simulink model "servo_real"  (Simulink 6.2)
settings: Solver=ode45  StartTime=0.0  StopTime=10  RelTol=1e-3
PreLoadFcn:
  | init_servo
libraries: cstblocks x2, simulink x2
settings Model: Creator=f96to  LastModifiedBy=toivo  ExtModeAutoUpdateStatusClock=off
settings OptimizationCC: BlockReduction=off  BooleanDataType=off
settings HardwareCC: TargetUnknown=on

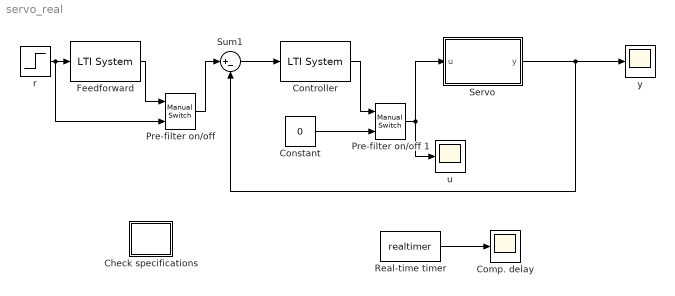
== system servo_real ==
  Check specifications : Subsystem
      settings: OpenFcn=specs_real
  Comp. delay : Scope
      settings: YMin=-0.5  YMax=1  SaveName=ScopeData2
  Constant : Constant  Value=0
  Controller : cstblocks/LTI System  sys=C  IC=[]
  Feedforward : cstblocks/LTI System  sys=F  IC=[]
  "Pre-filter on/off " : simulink/Signal Routing/Manual Switch  sw=0  action=0
  Pre-filter on/off 1 : simulink/Signal Routing/Manual Switch  sw=1  action=0
  Real-time timer : S-Function  FunctionName=realtimer  Parameters=0.01
  Servo : Subsystem
  Sum1 : Sum  Inputs=|+-  SaturateOnIntegerOverflow=on  InputSameDT=on
  r : Step  After=8  SampleTime=0
  u : Scope
      settings: YMin=-1  YMax=1  SaveName=u_out_real
  y : Scope
      settings: TimeRange=10  YMin=0  YMax=10  SaveName=y_out_real
  wires:
  Sum1/1 -> Controller/1
  r/1 -> Feedforward/1, "Pre-filter on/off "/2
  Real-time timer/1 -> Comp. delay/1
  Servo/1(y) -> y/1, Sum1/2
  "Pre-filter on/off "/1 -> Sum1/1
  Feedforward/1 -> "Pre-filter on/off "/1
  Constant/1 -> Pre-filter on/off 1/2
  Pre-filter on/off 1/1 -> Servo/1(u), u/1
  Controller/1 -> Pre-filter on/off 1/1

== system servo_real/Check specifications ==

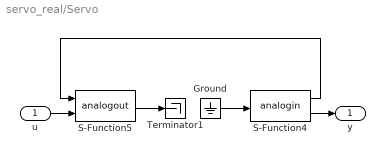
== system servo_real/Servo ==
  u : Inport  Port=1  LatchInput=off
  Ground : Ground
  S-Function4 : S-Function  FunctionName=analogin  Parameters=0.01 [1]
  S-Function5 : S-Function  FunctionName=analogout  Parameters=0.01 [0]
  Terminator1 : Terminator
  y : Outport
  wires:
  Ground/1 -> S-Function4/1
  S-Function5/1 -> Terminator1/1
  S-Function4/1 -> S-Function5/1
  S-Function4/2 -> y/1
  u/1 -> S-Function5/2
